simulink model "Zadanie_4"  (Simulink 7.1)
settings: Solver=ode45  StartTime=0.0  StopTime=4000  RelTol=1e-3
settings Model: Creator=Michal  LastModifiedBy=Michal

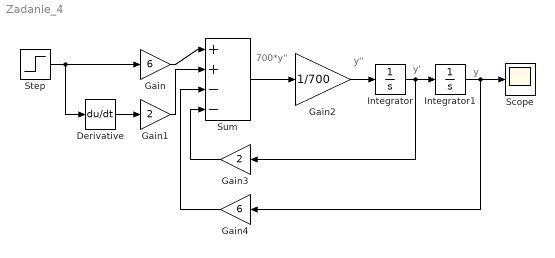
== system Zadanie_4 ==
  note: 700*y''
  note: y''
  note: y'
  note: y
  Derivative : Derivative
  Gain : Gain  Gain=6  ParameterDataType=sfix(16)  ParameterScaling=2^0  OutDataType=sfix(16)  OutScaling=2^0
  Gain1 : Gain  Gain=2  ParameterDataType=sfix(16)  ParameterScaling=2^0  OutDataType=sfix(16)  OutScaling=2^0
  Gain2 : Gain  Gain=1/700  ParameterDataType=sfix(16)  ParameterScaling=2^0  OutDataType=sfix(16)  OutScaling=2^0
  Gain3 : Gain  Orientation=left  Gain=2  ParameterDataType=sfix(16)  ParameterScaling=2^0  OutDataType=sfix(16)  OutScaling=2^0
  Gain4 : Gain  Orientation=left  Gain=6  ParameterDataType=sfix(16)  ParameterScaling=2^0  OutDataType=sfix(16)  OutScaling=2^0
  Integrator : Integrator
  Integrator1 : Integrator
  Scope : Scope
  Step : Step  SampleTime=0
  Sum : Sum  Inputs=|++--  OutDataType=sfix(16)  OutScaling=2^0
  wires:
  Step/1 -> Gain/1, Derivative/1
  Derivative/1 -> Gain1/1
  Gain/1 -> Sum/1
  Gain1/1 -> Sum/2
  Sum/1 -> Gain2/1
  Gain2/1 -> Integrator/1
  Integrator/1 -> Integrator1/1, Gain3/1
  Integrator1/1 -> Scope/1, Gain4/1
  Gain3/1 -> Sum/4
  Gain4/1 -> Sum/3
